simulink model "assgn1_part2"  (R2023a)
settings: Solver=VariableStepAuto  StartTime=0.0  StopTime=0.3  RelTol=1e-3
values from neighbouring files (symbols this model uses):
  C = 1e-06    [variables.m]
  L = 0.01    [variables.m]
  R = 40    [variables.m]
settings Model: Creator=Anirvan Krishna  LastModifiedBy=Anirvan Krishna
settings DataIOCC: Refine=500

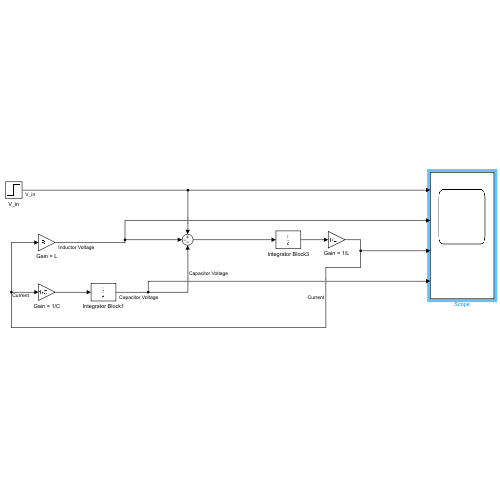
[thumbnail: Simulink's stored preview of the top-level diagram]
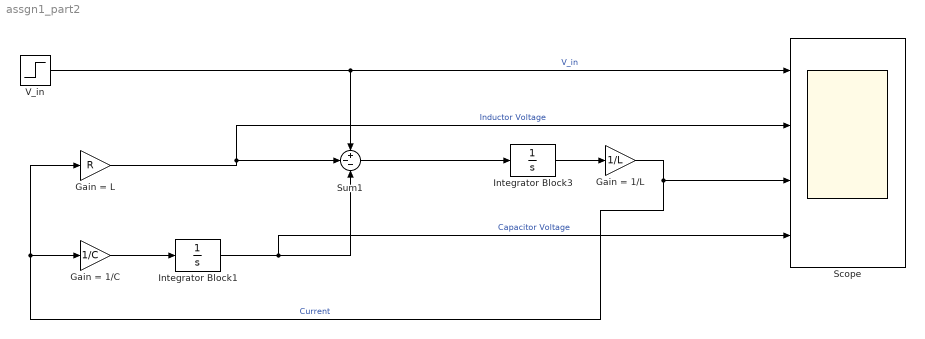
== system assgn1_part2 ==
  Gain = 1/C : Gain  Gain=1/C
  Gain = 1/L : Gain  Gain=1/L
  Gain = L : Gain  Gain=R
  Integrator Block1 : TransferFcn  Denominator=[1 0]
  Integrator Block3 : TransferFcn  Denominator=[1 0]
  Scope : Scope  NumInputPorts=4
  Sum1 : Sum  Inputs=+--
  V_in : Step  Time=0.2  SampleTime=0
  wires:
  Gain = L/1 -> Scope/2, Sum1/2  "Inductor Voltage"
  Gain = 1/C/1 -> Integrator Block1/1
  V_in/1 -> Scope/1, Sum1/1  "V_in"
  Sum1/1 -> Integrator Block3/1
  Gain = 1/L/1 -> Gain = 1/C/1, Gain = L/1, Scope/3  "Current"
  Integrator Block1/1 -> Scope/4, Sum1/3  "Capacitor Voltage"
  Integrator Block3/1 -> Gain = 1/L/1
